simulink model "atmosphere_blank_model"  (R2024b)
settings: Solver=VariableStepAuto  StartTime=0.0  StopTime=10.0  RelTol=1e-3
libraries: atmospheree x2
settings Model: Creator=user  LastModifiedBy=user

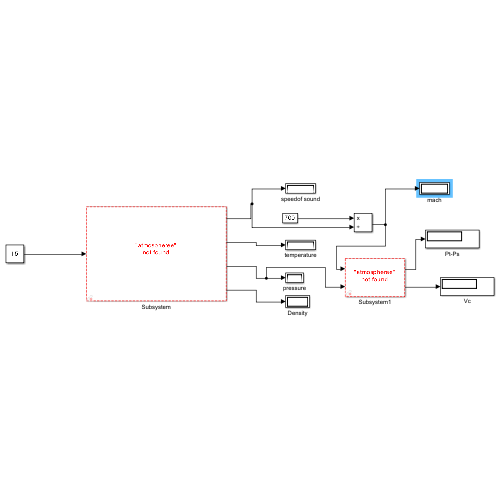
[thumbnail: Simulink's stored preview of the top-level diagram]
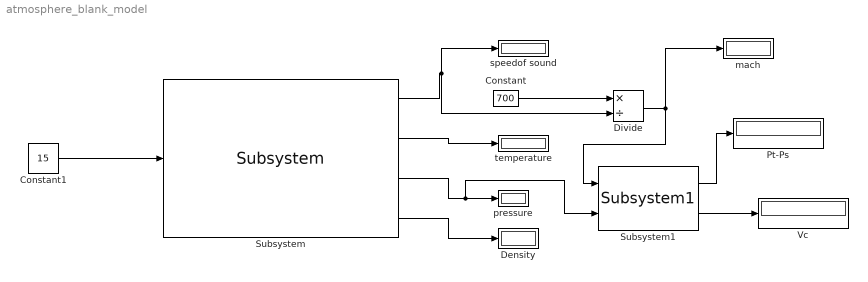
== system atmosphere_blank_model ==
  Constant : Constant  Value=700
  Constant1 : Constant  Value=15
  Density : Display
  Divide : Product  Inputs=*/
  Pt-Ps : Display
  Subsystem : atmospheree/Subsystem/Subsystem  SystemSampleTime=-1  VariantActivationTime=update diagram  AllowFlexibleInterface=on  Latency=0  AutoFrameSizeCalculation=off
  Subsystem1 : atmospheree/Subsystem/Subsystem1  SystemSampleTime=-1  VariantActivationTime=update diagram  AllowFlexibleInterface=on  Latency=0  AutoFrameSizeCalculation=off
  Vc : Display
  mach : Display
  pressure : Display
  speedof sound : Display
  temperature : Display
  wires:
  Subsystem/3 -> pressure/1, Subsystem1/2
  Subsystem/2 -> temperature/1
  Constant1/1 -> Subsystem/1
  Subsystem/1 -> speedof sound/1, Divide/2
  Subsystem1/1 -> Pt-Ps/1
  Divide/1 -> mach/1, Subsystem1/1
  Constant/1 -> Divide/1
  Subsystem/4 -> Density/1
  Subsystem1/2 -> Vc/1
